simulink model "ExperimentalCarrier"  (R2015b)
settings: Solver=ode45  StartTime=0.0  StopTime=60  FixedStep=0.001  RelTol=1e-4
model workspace (MAT data in the model file):
  CX = [-0.0973267994662 -0.079334770792 -0.063312708602 -0.0492783817904 -0.0372483838751 -0.0272381795582 -0.0192622767468 -0.0133348794834 -0.00947247058383 -0.00770460619817 -0.00779177365154 -0.010332184952 ... (651 elements, 31x21)]
  CX_P = [0.00223913348595 0.00226279846593 0.00215584206323 0.00191826427785 0.0015500651098 0.00105124455907 0.000421802625665 -0.000338260690416 -0.00122894538917 -0.00225025147061 -0.00340217893471 -0.0046847277815 ... (651 elements, 31x21)]
  CX_Q = [0.566750126524 0.513799273419 0.46074149597 0.407560115115 0.354235092058 0.300738098816 0.247021798665 0.193002362465 0.138579422321 0.0841448328254 0.0156800910173 -0.028587220216 ... (651 elements, 31x21)]
  CX_R = [0.00872473439328 0.00961108484928 0.0104908055113 0.0113660862689 0.0122394567236 0.0131139410899 0.0139934759578 0.0148843304351 0.0158005787982 0.0167844985256 0.0173214701743 0.0192824833308 ... (651 elements, 31x21)]
  CX_d_elevator = [0.029681120923 0.0264274948833 0.0231424780296 0.019826833889 0.0164811360769 0.0131055318554 0.00969907215747 0.00625794011772 0.00277062099267 -0.000820697586383 -0.00752061307428 -0.00815142995882 ... (651 elements, 31x21)]
  CX_d_rudder = [-0.00683814731464 -0.00579287968011 -0.00473313798197 -0.00365917618136 -0.00257115069818 -0.00146908461552 -0.000352779652782 0.000778396676178 0.0019254949791 0.00307845824922 0.00430777388103 0.00587395376473 ... (651 elements, 31x21)]
  CY = [0.0748502535538 0.0755645920384 0.0762601803819 0.076936530444 0.0775935707011 0.0782321665355 0.078855460083 0.0794722913019 0.0801051244106 0.0807983900173 0.0815089407636 0.0810999911453 ... (651 elements, 31x21)]
  CY_P = [0.314314541533 0.314908852342 0.315908686179 0.317314043043 0.319124922936 0.321341325856 0.323963251804 0.32699070078 0.330423672784 0.334262167815 0.338506185874 0.343155726961 ... (651 elements, 31x21)]
  CY_Q = [0.206845108985 0.212153285689 0.217549246201 0.223041221006 0.22863865097 0.234352353828 0.240194164072 0.246174375163 0.252295596359 0.258590970539 0.26593702078 0.276814416222 ... (651 elements, 31x21)]
  CY_R = [-0.299983586918 -0.303050767939 -0.30608450573 -0.309088417238 -0.312066630946 -0.315024477354 -0.317970440697 -0.320921537604 -0.323916102322 -0.327010675103 -0.329661903523 -0.331314720608 ... (651 elements, 31x21)]
  CY_d_elevator = [0.0241602483601 0.024862141616 0.0255735782381 0.0262950172254 0.0270270636195 0.0277705820366 0.0285269750226 0.0292988478742 0.0300914026037 0.030913435532 0.0317596917419 0.0324941126108 ... (651 elements, 31x21)]
  CY_d_rudder = [-0.129392052709 -0.131156233114 -0.132888496587 -0.13458992916 -0.13626179938 -0.137905650351 -0.139523580046 -0.141119005177 -0.142698155317 -0.144262742569 -0.145575423934 -0.146927528452 ... (651 elements, 31x21)]
  CZ = [-0.635288026255 -0.561513437672 -0.486937541039 -0.411613157493 -0.335593450001 -0.258932000134 -0.181683022099 -0.10390236702 -0.025657439009 0.0528154193638 0.128636653723 0.209168379022 ... (651 elements, 31x21)]
  CZ_P = [-0.0426180741921 -0.040371283283 -0.0379977363135 -0.0354974332835 -0.0328703741931 -0.0301165590423 -0.027235987831 -0.0242286605594 -0.0210945772272 -0.0178337378347 -0.0144461423817 -0.0109317908683 ... (651 elements, 31x21)]
  CZ_Q = [6.96025865077 6.98114129849 7.00206820292 7.02304903766 7.04409127039 7.06519952703 7.08637371713 7.10760603499 7.12891815552 7.15129935899 7.15392062661 7.18837906802 ... (651 elements, 31x21)]
  CZ_R = [-0.105405414656 -0.106545289739 -0.107737293614 -0.108987554898 -0.110302712806 -0.111690005069 -0.113157533015 -0.114714527104 -0.116362189514 -0.11786971515 -0.114666901886 -0.118318379275 ... (651 elements, 31x21)]
  CZ_d_elevator = [0.51008994796 0.512918903365 0.515635142398 0.518238988463 0.520730557555 0.523109824579 0.525376856974 0.527532585768 0.529582683355 0.53158310039 0.53222009415 0.532991323176 ... (651 elements, 31x21)]
  CZ_d_rudder = [-0.0994246348718 -0.101114338005 -0.102795749856 -0.104468657243 -0.106132886268 -0.107788391525 -0.109435540346 -0.111075916846 -0.112714334729 -0.114363388416 -0.115472857798 -0.116943666826 ... (651 elements, 31x21)]
  Cl = [-0.0385814765962 -0.0383389644596 -0.0380848835968 -0.0378195009591 -0.0375431159662 -0.0372560730473 -0.0369588021987 -0.0366519368415 -0.0363364206354 -0.0360097812088 -0.0355885143095 -0.0352015390645 ... (651 elements, 31x21)]
  Cl_P = [-0.410096776624 -0.411715869817 -0.413321511523 -0.414913701743 -0.416492440476 -0.418057727723 -0.419609563483 -0.421147947757 -0.422672880544 -0.424184361845 -0.425682391659 -0.427166969987 ... (651 elements, 31x21)]
  Cl_Q = [0.0121734873015 0.0115511634771 0.0109219874117 0.0102856172191 0.00964162351347 0.00898936687588 0.00832771640535 0.00765433243871 0.00696211625156 0.00619409954578 0.00511750960358 0.00438446572798 ... (651 elements, 31x21)]
  Cl_R = [0.0639194118456 0.0641980766094 0.0644722880685 0.0647423901469 0.0650087480028 0.0652717875848 0.0655321272397 0.0657909713502 0.0660509927516 0.066314134037 0.0664428977346 0.0665956593355 ... (651 elements, 31x21)]
  Cl_d_elevator = [-0.00083845092376 -0.000897333841468 -0.000957239499541 -0.00101816580014 -0.00108011314323 -0.00114310126406 -0.00120721661945 -0.00127274325287 -0.00134057483614 -0.00141463059496 -0.00150116458646 -0.00150417720092 ... (651 elements, 31x21)]
  Cl_d_rudder = [0.0120074370195 0.0121224981409 0.0122343776715 0.0123431699853 0.0124489831282 0.0125519544191 0.0126522973225 0.0127504304685 0.0128472820476 0.012944583953 0.0130167454048 0.0130728202844 ... (651 elements, 31x21)]
  Cm = [0.0973465601848 0.0882383997807 0.0791321401801 0.0700083578182 0.060846163509 0.0516235998805 0.0423185376691 0.03291173616 0.0234098703618 0.0141912971055 0.0115389891247 -0.00108731819606 ... (651 elements, 31x21)]
  Cm_P = [0.204940910369 0.202805913545 0.20033190145 0.197518874086 0.194366831451 0.190875773546 0.187045700371 0.182876611925 0.17836850821 0.173521389224 0.168335254967 0.162810105441 ... (651 elements, 31x21)]
  Cm_Q = [-8.8302811579 -8.84673802608 -8.86380445529 -8.8815160128 -8.89990381522 -8.91899396376 -8.93880586357 -8.95935222087 -8.98073821097 -9.00528706826 -8.98625605481 -9.03648930164 ... (651 elements, 31x21)]
  Cm_R = [0.231203964913 0.23319997533 0.235299090374 0.237514849258 0.239861907942 0.242356170567 0.245015146547 0.247857975971 0.250885037596 0.253592063858 0.24580144055 0.252971901877 ... (651 elements, 31x21)]
  Cm_d_elevator = [-1.16934045694 -1.17556162403 -1.1814926709 -1.18713462751 -1.19248809506 -1.19755345312 -1.20233156667 -1.2068260282 -1.21105317786 -1.21514844284 -1.21623242778 -1.21673947768 ... (651 elements, 31x21)]
  Cm_d_rudder = [0.221327907125 0.224938352672 0.228521302045 0.232076418337 0.235603478751 0.239102604189 0.24257498777 0.246024952347 0.249465016904 0.252925369172 0.255135515483 0.258069205799 ... (651 elements, 31x21)]
  Cn = [0.0239084920706 0.0233651881183 0.0228219583067 0.0222793256831 0.0217379864069 0.0211990203144 0.0206644263801 0.0201384574022 0.0196305829364 0.0191582088364 0.0187126782059 0.0177875778536 ... (651 elements, 31x21)]
  Cn_P = [0.00271348744888 0.000830692215513 -0.000879092281498 -0.00241586604216 -0.00377962906647 -0.00497038135443 -0.00598812290603 -0.00683285372129 -0.0075045738002 -0.00800328314275 -0.00832898174895 -0.0084816696188 ... (651 elements, 31x21)]
  Cn_Q = [0.0646895607463 0.0668587351559 0.0690696353792 0.0713263026419 0.0736328941188 0.0759930959236 0.078408543068 0.0808750323066 0.0833760949483 0.0858871158776 0.0879312223138 0.0933690960242 ... (651 elements, 31x21)]
  Cn_R = [-0.107505906228 -0.108368888514 -0.109223762874 -0.110071896296 -0.110914888897 -0.111754897972 -0.112595502998 -0.113443913399 -0.114315599189 -0.115230945783 -0.115971844659 -0.116177724127 ... (651 elements, 31x21)]
  Cn_d_elevator = [0.00836627067687 0.00863561072168 0.00890974810625 0.00918895143726 0.009473528048 0.00976381947702 0.0100601758992 0.0103628424776 0.0106713097064 0.0109780163579 0.011109463637 0.0115746093706 ... (651 elements, 31x21)]
  Cn_d_rudder = [-0.0546400598137 -0.0553510121202 -0.0560495856635 -0.0567362885882 -0.0574116958811 -0.0580764807608 -0.0587315154598 -0.0593781486964 -0.060018716409 -0.060653217797 -0.0611661774955 -0.061673059209 ... (651 elements, 31x21)]
  aircraft_geometry_name = 'ExperimentalCarrier'
  alpha = [-0.174532925199 -0.157079632679 -0.13962634016 -0.12217304764 -0.10471975512 -0.0872664625997 -0.0698131700798 -0.0523598775598 -0.0349065850399 -0.0174532925199 0 0.0174532925199 ... (31 elements, 31x1)]
  beta = [-0.174532925199 -0.157079632679 -0.13962634016 -0.12217304764 -0.10471975512 -0.0872664625997 -0.0698131700798 -0.0523598775598 -0.0349065850399 -0.0174532925199 0 0.0174532925199 ... (21 elements, 21x1)]
  centerOfGravity = -0.092
  mass = 1.56
  mean_chord = 0.25
  spanwidth = 1.5
undefined symbols (not defined in the file): Earth, WGS84
libraries: aerolibconvert2 x6, aerolibnav x3, aerolibasang x2, aerolibfltsims x2, aerolib6dof2 x1, aerolibadyn x1, aerolibtransform2 x1, aerolibanimutils x1, aerolibatmos2 x1, aerolibgravity2 x1
(part 2 of 2)

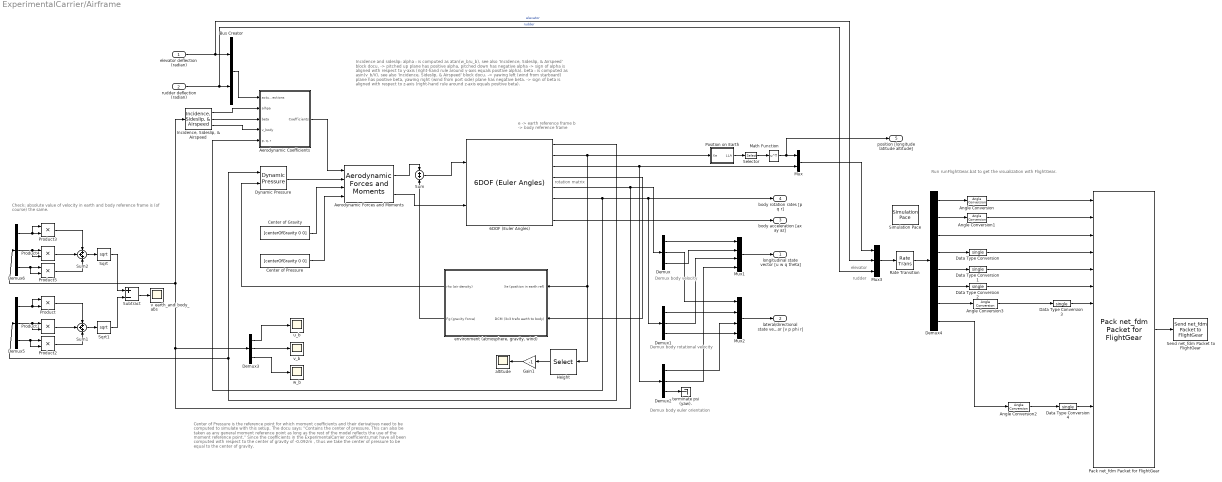
== system ExperimentalCarrier/Airframe ==
  note: rotation matrix
  note: Check: absolute value of velocity in earth and body reference frame is
      | (of course) the same.
  note: rudder
  note: elevator
  note: Incidence and sideslip:
      | alpha : is computed as atan(w_b/u_b), see also 'Incidence, Sideslip, & Airspeed' block docu.
      | -> pitched up plane has positive alpha, pitched down has negative alpha
      | -> sign of alpha is aligned with respect to y-axis (right-hand rule around y-axis equals positive alpha).
      | beta : is computed as asin(v_b/V), see also 'Incidence, Sideslip, & Airspeed' block docu.
      | -> yawing left (wind from starboard) plane has positive beta, yawing right (wind from port side) plane has negative beta.
      | -> sign of beta is aligned with respect to z-axis (right-hand rule around z-axis equals positive beta).
  note: Demux body velocity
  note: Run runFlightGear.bat to get the visualization with FlightGear.
  note: e -> earth reference frame
      | b -> body reference frame
  note: Center of Pressure is the reference point for which moment coefficients and their derivatives need to be computed to simulate with this setup.
      | The docu says: "Contains the center of pressure. This can also be taken as any general moment reference point as long as the rest of the model
      | reflects the use of the moment reference point." Since the coefficients in the ExperimentalCarrier coefficients.mat have all been computed with respect to
      | the center of gravity of -0.092m , thus we take the center of pressure to be equal to the center of gravity.
  note: Demux body rotational velocity
  note: Demux body euler orientation
  elevator deflection (radian) : Inport
  rudder deflection (radian) : Inport  Port=2
  6DOF (Euler Angles) : aerolib6dof2/6DOF (Euler Angles)  units=Metric (MKS)  mtype=Fixed  rep=Euler Angles  xme_0=[-12071.91150883141;0;-800.0]  Vm_0=[11 0 0]  eul_0=[0 -1.2 0]  pm_0=[0 0 0]  mass_0=mass  mass_e=0.5  mass_f=2.0  inertia=eye(3)  inertia_e=eye(3)  inertia_f=2*eye(3)  k_quat=1.0  vre_flag=on
  "Aerodynamic Forces and Moments " : aerolibadyn/Aerodynamic Forces and Moments   inputAxes=Body  outputForceAxes=Body  outputMomentAxes=Body  S=spanwidth*mean_chord  b=spanwidth  cbar=mean_chord
  Aerodynamic Coefficients : Subsystem
  Angle Conversion : aerolibconvert2/Angle Conversion  IU=deg  OU=rad
  Angle Conversion1 : aerolibconvert2/Angle Conversion  IU=deg  OU=rad
  Angle Conversion2 : aerolibconvert2/Angle Conversion  IU=rad  OU=deg
  Angle Conversion3 : aerolibconvert2/Angle Conversion  IU=rad  OU=deg
  Bus Creator : BusCreator  Inputs=2
  Center of Gravity : Constant  Value=[centerOfGravity 0 0]
  Center of Pressure : Constant  Value=[centerOfGravity 0 0]
  Data Type Conversion{,1..4} (5 alike) : DataTypeConversion  OutDataTypeStr=single
  Demux{,1..3,5..6} (6 alike) : Demux  Outputs=3
  Demux4 : Demux  Outputs=8
  Dynamic Pressure : aerolibasang/Dynamic Pressure
  Gain1 : Gain  Gain=-1
  Height : Selector  InputPortWidth=3  IndexOptions=Index vector (dialog)  Indices=[3]  OutputSizes=1
  "Incidence, Sideslip, & Airspeed" : aerolibasang/Incidence, Sideslip, & Airspeed
  Math Function : Math  Operator=transpose  SaturateOnIntegerOverflow=on
  Mux : Mux  Inputs=2
  Mux1 : Mux
  Mux2 : Mux
  Mux3 : Mux  Inputs=3
  Pack net_fdm Packet for FlightGear : aerolibfltsims/Pack net_fdm Packet for FlightGear  FlightGearVersion=v3.4  ShowPositionAttitudeInputs=on  ShowVelocityAccelerationInputs=off  ShowControlSurfacePositionInputs=on  ShowEngineFuelInputs=off  ShowLandingGearInputs=off  ShowEnvironmentInputs=off  SampleTime=1/30
  Position on Earth : Subsystem  Priority=1  TreatAsAtomicUnit=on
  Product{,1..5} (6 alike) : Product  RndMeth=Zero
  Rate Transition : RateTransition  Integrity=off  OutPortSampleTime=1/30
  Selector : Selector  InputPortWidth=3  IndexOptions=Index vector (dialog)  Indices=[2 1 3]  OutputSizes=1
  Send net_fdm Packet to FlightGear : aerolibfltsims/Send net_fdm Packet to FlightGear  DestinationIpAddress=127.0.0.1  DestinationPort=5502  LocalIpPort=-1  varLen=off  SampleTime=1/30
  Simulation Pace : aerolibanimutils/Simulation Pace  SimulationPace=1  SleepMode=MATLAB Thread  OutputPaceError=off  SampleTime=1/30
      settings: AttributesFormatString=%<SimulationPace> sec/sec
  Sqrt : Sqrt  SaturateOnIntegerOverflow=on
  Sqrt1 : Sqrt  SaturateOnIntegerOverflow=on
  Subtract : Sum  Inputs=+-
  Sum : Sum
  Sum1 : Sum  Inputs=+++
  Sum2 : Sum  Inputs=+++
  altitude : Scope
  "environment (atmosphere, gravity, wind)" : Subsystem
  terminate psi (yaw). : Terminator
  u_b : Scope
  v_b : Scope
  v_earth_and_body_abs : Scope
  w_b : Scope
  longitudinal state vector [u w q theta] : Outport
  lateral/directional state vector [v p phi r] : Outport  Port=2
  body acceleration [ax ay az] : Outport  Port=3
  body rotation rates [p q r] : Outport  Port=4
  position [longitude latitude altitude] : Outport  Port=5
  wires:
  "Aerodynamic Forces and Moments "/1 -> Sum/1
  "Aerodynamic Forces and Moments "/2 -> 6DOF (Euler Angles)/2
  Center of Gravity/1 -> "Aerodynamic Forces and Moments "/3
  Center of Pressure/1 -> "Aerodynamic Forces and Moments "/4
  Dynamic Pressure/1 -> "Aerodynamic Forces and Moments "/2
  6DOF (Euler Angles)/1 -> Dynamic Pressure/1, Demux5/1
  6DOF (Euler Angles)/2 -> Height/1, "environment (atmosphere, gravity, wind)"/1(Xe (position in earth ref)), Position on Earth/1(Xe)
  Position on Earth/1(LLA) -> Selector/1
  6DOF (Euler Angles)/4 -> "environment (atmosphere, gravity, wind)"/2(DCM (3x3 trafo earth to body))
  6DOF (Euler Angles)/3 -> Mux/2, Demux2/1
  6DOF (Euler Angles)/5 -> "Incidence, Sideslip, & Airspeed"/1, Demux6/1, Demux3/1, Demux/1
  6DOF (Euler Angles)/6 -> Aerodynamic Coefficients/5("p, q, r"), body rotation rates [p q r]/1, Demux1/1
  Math Function/1 -> position [longitude latitude altitude]/1, Mux/1
  Mux/1 -> Mux3/1
  Selector/1 -> Math Function/1
  "environment (atmosphere, gravity, wind)"/1(rho (air density)) -> Dynamic Pressure/2
  "environment (atmosphere, gravity, wind)"/2(Fg (gravity force)) -> Sum/2
  Height/1 -> Gain1/1
  "Incidence, Sideslip, & Airspeed"/1 -> Aerodynamic Coefficients/2(alhpa)
  "Incidence, Sideslip, & Airspeed"/2 -> Aerodynamic Coefficients/3(beta)
  "Incidence, Sideslip, & Airspeed"/3 -> Aerodynamic Coefficients/4(v_body)
  Aerodynamic Coefficients/1(Coefficients) -> "Aerodynamic Forces and Moments "/1
  Gain1/1 -> altitude/1
  Bus Creator/1 -> Aerodynamic Coefficients/1(actuator deflections)
  elevator deflection (radian)/1 -> Mux3/2, Bus Creator/1  "elevator"
  rudder deflection (radian)/1 -> Mux3/3, Bus Creator/2  "rudder"
  Sum/1 -> 6DOF (Euler Angles)/1
  Demux/1 -> Mux1/1
  Demux/3 -> Mux1/2
  Demux/2 -> Mux2/1
  Demux1/2 -> Mux1/3
  Demux1/1 -> Mux2/2
  Demux1/3 -> Mux2/4
  Demux2/1 -> Mux2/3
  Demux2/2 -> Mux1/4
  Demux2/3 -> terminate psi (yaw)./1
  Mux2/1 -> lateral/directional state vector [v p phi r]/1
  Mux1/1 -> longitudinal state vector [u w q theta]/1
  Demux3/1 -> u_b/1
  Demux3/2 -> v_b/1
  Demux3/3 -> w_b/1
  Pack net_fdm Packet for FlightGear/1 -> Send net_fdm Packet to FlightGear/1
  Demux4/1 -> Angle Conversion/1
  Demux4/2 -> Angle Conversion1/1
  Demux4/3 -> Pack net_fdm Packet for FlightGear/3
  Demux4/4 -> Data Type Conversion/1
  Demux4/5 -> Data Type Conversion1/1
  Demux4/6 -> Data Type Conversion2/1
  Rate Transition/1 -> Demux4/1
  Angle Conversion/1 -> Pack net_fdm Packet for FlightGear/1
  Angle Conversion1/1 -> Pack net_fdm Packet for FlightGear/2
  Data Type Conversion/1 -> Pack net_fdm Packet for FlightGear/4
  Data Type Conversion1/1 -> Pack net_fdm Packet for FlightGear/5
  Data Type Conversion2/1 -> Pack net_fdm Packet for FlightGear/6
  Mux3/1 -> Rate Transition/1
  Demux4/7 -> Angle Conversion3/1
  Demux4/8 -> Angle Conversion2/1
  Data Type Conversion3/1 -> Pack net_fdm Packet for FlightGear/7
  Data Type Conversion4/1 -> Pack net_fdm Packet for FlightGear/13
  Angle Conversion2/1 -> Data Type Conversion4/1
  Angle Conversion3/1 -> Data Type Conversion3/1
  Product2/1 -> Sum1/3
  Demux5/3 -> Product2/2, Product2/1
  Product/1 -> Sum1/1
  Product1/1 -> Sum1/2
  Sum1/1 -> Sqrt1/1
  Demux5/1 -> Product/2, Product/1
  Demux5/2 -> Product1/1, Product1/2
  Product5/1 -> Sum2/3
  Demux6/3 -> Product5/2, Product5/1
  Product3/1 -> Sum2/1
  Product4/1 -> Sum2/2
  Sum2/1 -> Sqrt/1
  Demux6/1 -> Product3/2, Product3/1
  Demux6/2 -> Product4/1, Product4/2
  Sqrt/1 -> Subtract/1
  Sqrt1/1 -> Subtract/2
  Subtract/1 -> v_earth_and_body_abs/1
  6DOF (Euler Angles)/8 -> body acceleration [ax ay az]/1

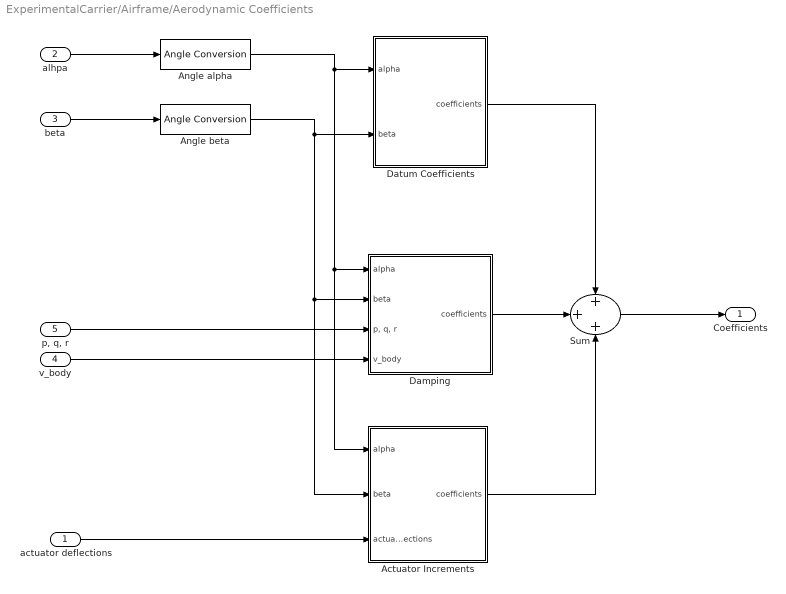
== system ExperimentalCarrier/Airframe/Aerodynamic Coefficients ==
  actuator deflections : Inport
  alhpa : Inport  Port=2
  beta : Inport  Port=3
  v_body : Inport  Port=4
  "p, q, r" : Inport  Port=5
  Actuator Increments : Subsystem
  Angle alpha : aerolibconvert2/Angle Conversion  IU=rad  OU=deg
  Angle beta : aerolibconvert2/Angle Conversion  IU=rad  OU=deg
  Damping : Subsystem
  Datum Coefficients : Subsystem
  Sum : Sum  Inputs=+++
  Coefficients : Outport
  wires:
  alhpa/1 -> Angle alpha/1
  Angle alpha/1 -> Actuator Increments/1(alpha), Damping/1(alpha), Datum Coefficients/1(alpha)
  Angle beta/1 -> Actuator Increments/2(beta), Damping/2(beta), Datum Coefficients/2(beta)
  Datum Coefficients/1(coefficients) -> Sum/1
  "p, q, r"/1 -> Damping/3("p, q, r")
  Damping/1(coefficients) -> Sum/2
  Sum/1 -> Coefficients/1
  v_body/1 -> Damping/4(v_body)
  beta/1 -> Angle beta/1
  actuator deflections/1 -> Actuator Increments/3(actuator deflections)
  Actuator Increments/1(coefficients) -> Sum/3

== system ExperimentalCarrier/Airframe/Position on Earth ==
  Xe : Inport
  Flat Earth to LLA : aerolibtransform2/Flat Earth to LLA  units=Metric (MKS)  ptype=Earth (WGS84)  F=1/298.257223563  R=6378137  LL0=[37.628738616666666,-1.223933911333333e+02]  psi=0
  Mux : Mux  Inputs=2
  href : Constant  Value=300
  LLA : Outport
  wires:
  Mux/1 -> LLA/1
  Xe/1 -> Flat Earth to LLA/1
  Flat Earth to LLA/1 -> Mux/1
  Flat Earth to LLA/2 -> Mux/2
  href/1 -> Flat Earth to LLA/2

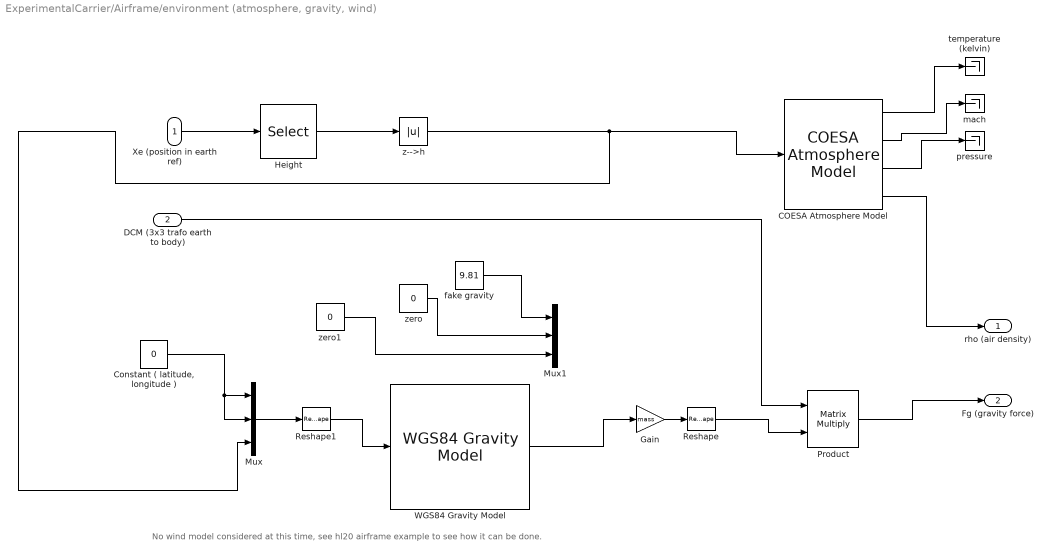
== system ExperimentalCarrier/Airframe/environment (atmosphere, gravity, wind) ==
  note: No wind model considered at this time, see hl20 airframe example to see how it can be done.
  Xe (position in earth ref) : Inport
  DCM (3x3 trafo earth to body) : Inport  Port=2
  COESA Atmosphere Model : aerolibatmos2/COESA Atmosphere Model  units=Metric (MKS)  spec=1976 COESA-extended U.S. Standard Atmosphere  model=Profile  profile_var=High temperature  profile_percent=1%  profile_alt=5 km (16404 ft)  envelope_var=High temperature  envelope_percent=1%  action=Warning
  "Constant ( latitude, longitude )" : Constant  Value=0
  Gain : Gain  Gain=mass
  Height : Selector  InputPortWidth=3  IndexOptions=Index vector (dialog)  Indices=[3]  OutputSizes=1
  Mux : Mux  Inputs=3
  Mux1 : Mux  Inputs=3
  Product : Product  Multiplication=Matrix(*)
  Reshape : Reshape
  Reshape1 : Reshape
  "WGS84 Gravity Model " : aerolibgravity2/WGS84 Gravity Model   model=WGS84 Taylor Series  units=Metric (MKS)  no_atmos=on  precessing=on  jd_loc=off  month=October  day=10  year=2004  no_centrifugal=on  action=Warning
  fake gravity : Constant  Value=9.81
  mach : Terminator
  pressure : Terminator
  temperature (kelvin) : Terminator
  z-->h : Abs  SaturateOnIntegerOverflow=on
  zero : Constant  Value=0
  zero1 : Constant  Value=0
  rho (air density) : Outport
  Fg (gravity force) : Outport  Port=2
  wires:
  Xe (position in earth ref)/1 -> Height/1
  Height/1 -> z-->h/1
  z-->h/1 -> Mux/3, COESA Atmosphere Model/1
  COESA Atmosphere Model/4 -> rho (air density)/1
  COESA Atmosphere Model/1 -> temperature (kelvin)/1
  COESA Atmosphere Model/2 -> mach/1
  COESA Atmosphere Model/3 -> pressure/1
  "Constant ( latitude, longitude )"/1 -> Mux/1, Mux/2
  Mux/1 -> Reshape1/1
  fake gravity/1 -> Mux1/1
  Gain/1 -> Reshape/1
  Reshape/1 -> Product/2
  DCM (3x3 trafo earth to body)/1 -> Product/1
  Product/1 -> Fg (gravity force)/1
  zero/1 -> Mux1/2
  zero1/1 -> Mux1/3
  Reshape1/1 -> "WGS84 Gravity Model "/1
  "WGS84 Gravity Model "/1 -> Gain/1

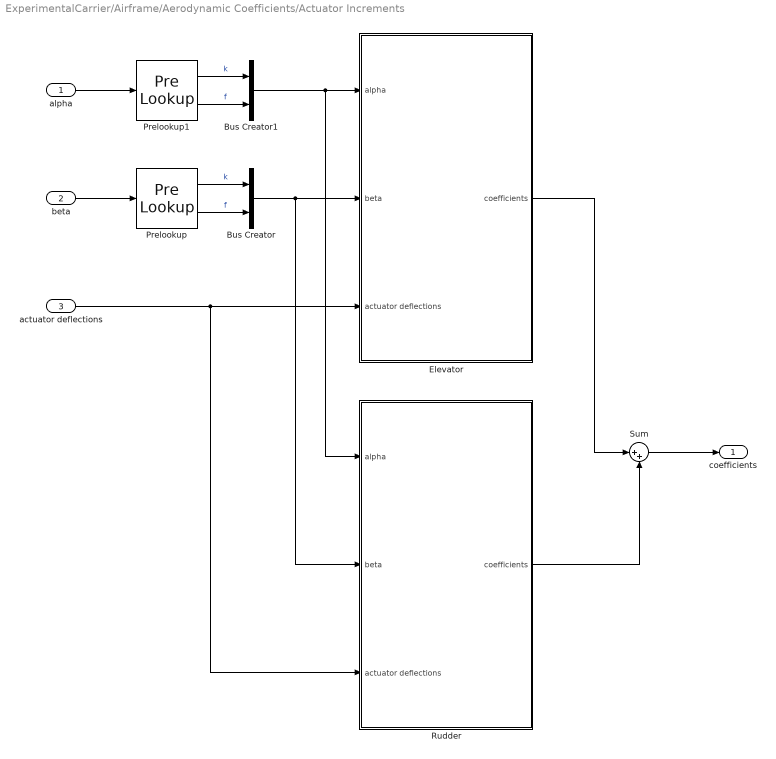
== system ExperimentalCarrier/Airframe/Aerodynamic Coefficients/Actuator Increments ==
  alpha : Inport
  beta : Inport  Port=2
  actuator deflections : Inport  Port=3
  Bus Creator : BusCreator  Inputs=2
  Bus Creator1 : BusCreator  Inputs=2
  Elevator : Subsystem
  Prelookup : PreLookup  BreakpointsData=beta*180/pi  ExtrapMethod=Linear
  Prelookup1 : PreLookup  BreakpointsData=alpha*180/pi  ExtrapMethod=Linear
  Rudder : Subsystem
  Sum : Sum  Inputs=|++
  coefficients : Outport
  wires:
  alpha/1 -> Prelookup1/1
  beta/1 -> Prelookup/1
  actuator deflections/1 -> Rudder/3(actuator deflections), Elevator/3(actuator deflections)
  Elevator/1(coefficients) -> Sum/1
  Sum/1 -> coefficients/1
  Bus Creator/1 -> Elevator/2(beta), Rudder/2(beta)
  Prelookup/1 -> Bus Creator/1  "k"
  Prelookup/2 -> Bus Creator/2  "f"
  Prelookup1/1 -> Bus Creator1/1  "k"
  Prelookup1/2 -> Bus Creator1/2  "f"
  Bus Creator1/1 -> Elevator/1(alpha), Rudder/1(alpha)
  Rudder/1(coefficients) -> Sum/2

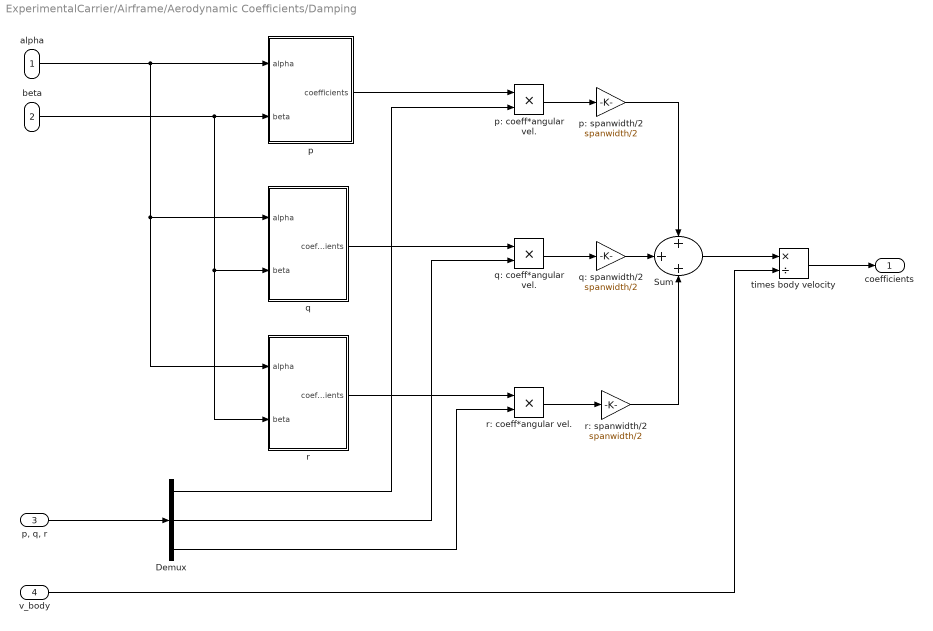
== system ExperimentalCarrier/Airframe/Aerodynamic Coefficients/Damping ==
  alpha : Inport
  beta : Inport  Port=2
  "p, q, r" : Inport  Port=3
  v_body : Inport  Port=4
  Demux : Demux  Outputs=3
  Sum : Sum  Inputs=+++
  p : Subsystem
  p: coeff*angular vel. : Product
  p: spanwidth/2 : Gain  Gain=spanwidth/2
  q : Subsystem
  q: coeff*angular vel. : Product
  q: spanwidth/2 : Gain  Gain=spanwidth/2
  r : Subsystem
  r: coeff*angular vel. : Product
  r: spanwidth/2 : Gain  Gain=spanwidth/2
  times body velocity : Product  Inputs=*/
  coefficients : Outport
  wires:
  alpha/1 -> r/1(alpha), q/1(alpha), p/1(alpha)
  beta/1 -> r/2(beta), q/2(beta), p/2(beta)
  p/1(coefficients) -> p: coeff*angular vel./1
  "p, q, r"/1 -> Demux/1
  p: coeff*angular vel./1 -> p: spanwidth/2/1
  p: spanwidth/2/1 -> Sum/1
  Sum/1 -> times body velocity/1
  v_body/1 -> times body velocity/2
  q/1(coefficients) -> q: coeff*angular vel./1
  r/1(coefficients) -> r: coeff*angular vel./1
  q: spanwidth/2/1 -> Sum/2
  r: spanwidth/2/1 -> Sum/3
  r: coeff*angular vel./1 -> r: spanwidth/2/1
  q: coeff*angular vel./1 -> q: spanwidth/2/1
  Demux/2 -> q: coeff*angular vel./2
  times body velocity/1 -> coefficients/1
  Demux/1 -> p: coeff*angular vel./2
  Demux/3 -> r: coeff*angular vel./2

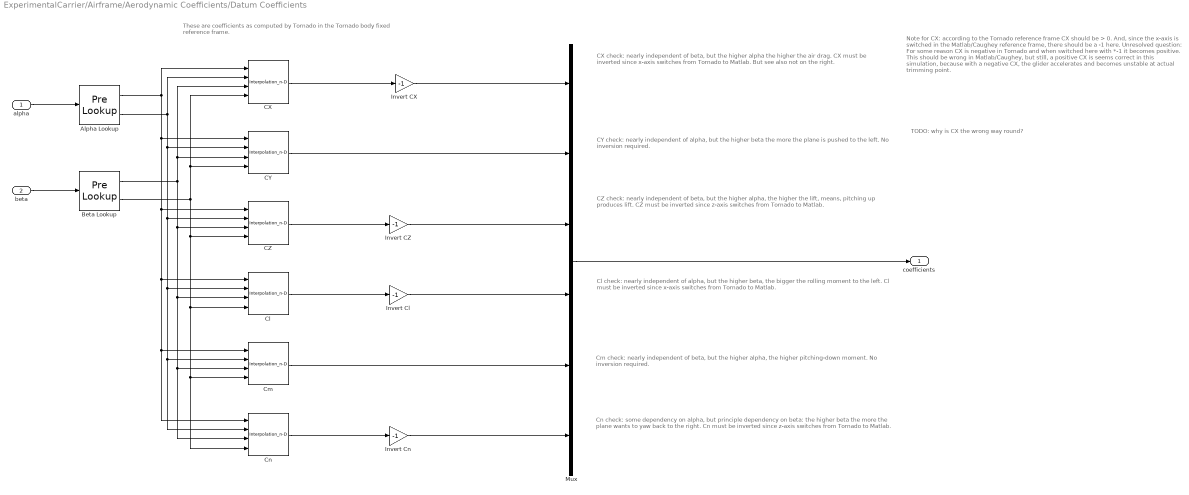
== system ExperimentalCarrier/Airframe/Aerodynamic Coefficients/Datum Coefficients ==
  note: Cl check: nearly independent of alpha, but the higher beta, the bigger the rolling moment to the left. Cl must be inverted since x-axis switches from Tornado to Matlab.
  note: CY check: nearly independent of alpha, but
      | the higher beta the more the plane is pushed to the left. No inversion required.
  note: These are coefficients as computed by Tornado in the
      | Tornado body fixed reference frame.
  note: Cm check: nearly independent of beta, but the higher alpha, the higher pitching-down moment. No inversion required.
  note: CZ check: nearly independent of beta, but the higher alpha, the higher the lift, means, pitching up produces lift. CZ must be inverted since z-axis switches from Tornado to Matlab.
  note: Note for CX: according to the Tornado reference frame
      | CX should be > 0. And, since the x-axis is switched in the
      | Matlab/Caughey reference frame, there should be a -1 here.
      | Unresolved question: For some reason CX is negative in Tornado
      | and when switched here with *-1 it becomes positive. This should
      | be wrong in Matlab/Caughey, but still, a positive CX is seems correct
      | in this simulation, because with a negative CX, the glider
      | accelerates and becomes unstable at actual trimming point.
  note: Cn check: some dependency on alpha, but principle dependency on beta: the higher beta the more the plane wants to yaw back to the right. Cn must be inverted since z-axis switches from Tornado to Matlab.
  note: CX check: nearly independent of beta, but the higher alpha the higher the air drag. CX must be inverted since x-axis switches from Tornado to Matlab. But see also not on the right.
  note: TODO:
      | why is CX the wrong way round?
  alpha : Inport
  beta : Inport  Port=2
  Alpha Lookup : PreLookup  BreakpointsData=alpha*180/pi  ExtrapMethod=Linear
  Beta Lookup : PreLookup  BreakpointsData=beta*180/pi  ExtrapMethod=Linear
  CX : Interpolation_n-D  Table=CX  InternalRulePriority=Speed
  CY : Interpolation_n-D  Table=CY  InternalRulePriority=Speed
  CZ : Interpolation_n-D  Table=CZ  InternalRulePriority=Speed
  Cl : Interpolation_n-D  Table=Cl  InternalRulePriority=Speed
  Cm : Interpolation_n-D  Table=Cm  InternalRulePriority=Speed
  Cn : Interpolation_n-D  Table=Cn  InternalRulePriority=Speed
  Invert CX : Gain  Gain=-1
  Invert CZ : Gain  Gain=-1
  Invert Cl : Gain  Gain=-1
  Invert Cn : Gain  Gain=-1
  Mux : Mux  Inputs=6
  coefficients : Outport
  wires:
  Alpha Lookup/1 -> Cl/1, Cm/1, Cn/1, CZ/1, CY/1, CX/1
  Alpha Lookup/2 -> Cm/2, Cn/2, Cl/2, CZ/2, CY/2, CX/2
  Beta Lookup/1 -> Cn/3, Cm/3, Cl/3, CZ/3, CX/3, CY/3
  Beta Lookup/2 -> Cm/4, Cn/4, Cl/4, CZ/4, CX/4, CY/4
  alpha/1 -> Alpha Lookup/1
  beta/1 -> Beta Lookup/1
  Mux/1 -> coefficients/1
  CZ/1 -> Invert CZ/1
  CY/1 -> Mux/2
  CX/1 -> Invert CX/1
  Cl/1 -> Invert Cl/1
  Cn/1 -> Invert Cn/1
  Invert CZ/1 -> Mux/3
  Invert Cl/1 -> Mux/4
  Invert Cn/1 -> Mux/6
  Invert CX/1 -> Mux/1
  Cm/1 -> Mux/5

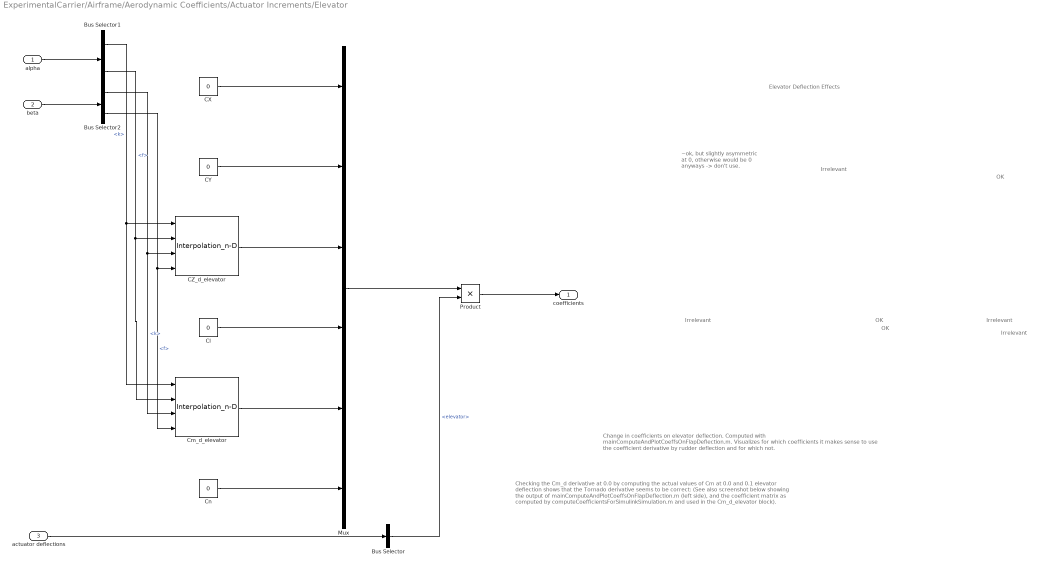
== system ExperimentalCarrier/Airframe/Aerodynamic Coefficients/Actuator Increments/Elevator ==
  note: Checking the Cm_d derivative at 0.0 by computing the actual values of Cm at 0.0 and 0.1 elevator deflection shows that the Tornado derivative seems to be correct:
      | (See also screenshot below showing the output of mainComputeAndPlotCoeffsOnFlapDeflection.m (left side), and the coefficient matrix as computed by computeCoefficientsForSimulinkSimulation.m and used in the Cm_d_elevator block).
  note: OK
  note: Irrelevant
  note: ~ok, but slightly
      | asymmetric at 0,
      | otherwise would
      | be 0 anyways
      | -> don't use.
  note: Irrelevant
  note: OK
  note: Irrelevant
  note: Change in coefficients on elevator deflection. Computed with mainComputeAndPlotCoeffsOnFlapDeflection.m.
      | Visualizes for which coefficients it makes sense to use the coefficient derivative by rudder deflection and for which not.
  note: Elevator Deflection Effects
  note: OK
  note: Irrelevant
  alpha : Inport
  beta : Inport  Port=2
  actuator deflections : Inport  Port=3
  Bus Selector : BusSelector  OutputSignals=elevator
  Bus Selector1 : BusSelector  OutputSignals=k,f
  Bus Selector2 : BusSelector  OutputSignals=k,f
  CX : Constant  Value=0
  CY : Constant  Value=0
  CZ_d_elevator : Interpolation_n-D  Table=CZ_d_elevator  InternalRulePriority=Speed
  Cl : Constant  Value=0
  Cm_d_elevator : Interpolation_n-D  Table=Cm_d_elevator  InternalRulePriority=Speed
  Cn : Constant  Value=0
  Mux : Mux  Inputs=6
  Product : Product
  coefficients : Outport
  wires:
  Bus Selector1/1 -> Cm_d_elevator/1, CZ_d_elevator/1  "<k>"
  Bus Selector1/2 -> Cm_d_elevator/2, CZ_d_elevator/2  "<f>"
  alpha/1 -> Bus Selector1/1
  Bus Selector2/1 -> Cm_d_elevator/3, CZ_d_elevator/3  "<k>"
  Bus Selector2/2 -> Cm_d_elevator/4, CZ_d_elevator/4  "<f>"
  CY/1 -> Mux/2
  CZ_d_elevator/1 -> Mux/3
  Cm_d_elevator/1 -> Mux/5
  actuator deflections/1 -> Bus Selector/1
  Product/1 -> coefficients/1
  Bus Selector/1 -> Product/2  "<elevator>"
  Mux/1 -> Product/1
  beta/1 -> Bus Selector2/1
  Cl/1 -> Mux/4
  Cn/1 -> Mux/6
  CX/1 -> Mux/1

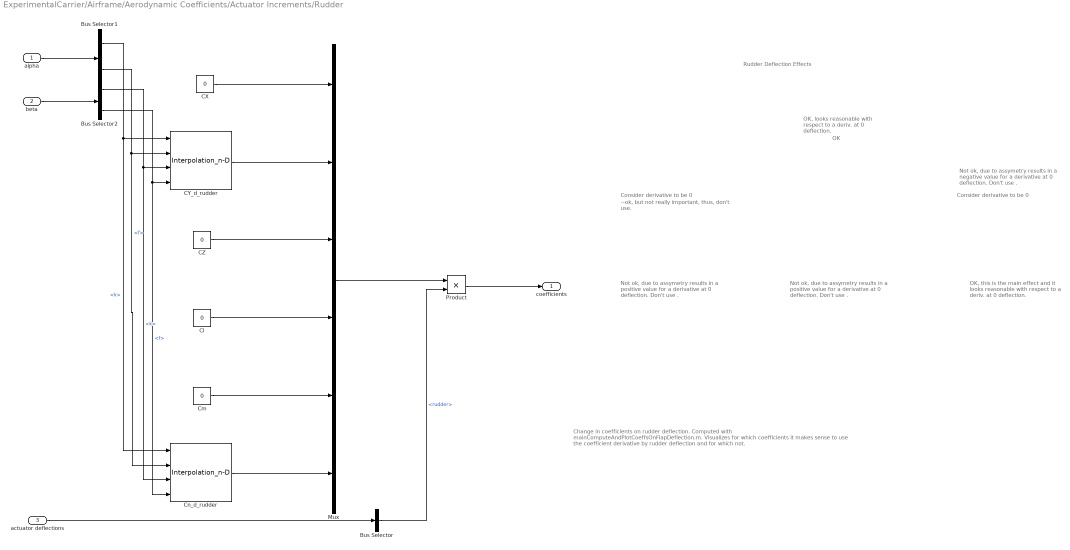
== system ExperimentalCarrier/Airframe/Aerodynamic Coefficients/Actuator Increments/Rudder ==
  note: Consider derivative to be 0
  note: Consider derivative to be 0
  note: OK
  note: Not ok, due to assymetry
      | results in a positive
      | value for a derivative at 0
      | deflection. Don't use .
  note: Not ok, due to assymetry
      | results in a positive
      | value for a derivative at 0
      | deflection. Don't use .
  note: OK, this is the main effect
      | and it looks reasonable
      | with respect to a deriv.
      | at 0 deflection.
  note: Not ok, due to assymetry
      | results in a negative
      | value for a derivative at 0
      | deflection. Don't use .
  note: OK, looks reasonable
      | with respect to a deriv.
      | at 0 deflection.
  note: ~ok, but not really important,
      | thus, don't use.
  note: Change in coefficients on rudder deflection. Computed with mainComputeAndPlotCoeffsOnFlapDeflection.m.
      | Visualizes for which coefficients it makes sense to use the coefficient derivative by rudder deflection and for which not.
  note: Rudder Deflection Effects
  alpha : Inport
  beta : Inport  Port=2
  actuator deflections : Inport  Port=3
  Bus Selector : BusSelector  OutputSignals=rudder
  Bus Selector1 : BusSelector  OutputSignals=k,f
  Bus Selector2 : BusSelector  OutputSignals=k,f
  CX : Constant  Value=0
  CY_d_rudder : Interpolation_n-D  Table=CY_d_rudder  InternalRulePriority=Speed
  CZ : Constant  Value=0
  Cl : Constant  Value=0
  Cm : Constant  Value=0
  Cn_d_rudder : Interpolation_n-D  Table=Cn_d_rudder  InternalRulePriority=Speed
  Mux : Mux  Inputs=6
  Product : Product
  coefficients : Outport
  wires:
  Bus Selector1/1 -> Cn_d_rudder/1, CY_d_rudder/1  "<k>"
  Bus Selector1/2 -> Cn_d_rudder/2, CY_d_rudder/2  "<f>"
  alpha/1 -> Bus Selector1/1
  Bus Selector2/1 -> Cn_d_rudder/3, CY_d_rudder/3  "<k>"
  Bus Selector2/2 -> Cn_d_rudder/4, CY_d_rudder/4  "<f>"
  CX/1 -> Mux/1
  CY_d_rudder/1 -> Mux/2
  CZ/1 -> Mux/3
  Cl/1 -> Mux/4
  Cn_d_rudder/1 -> Mux/6
  actuator deflections/1 -> Bus Selector/1
  Product/1 -> coefficients/1
  Bus Selector/1 -> Product/2  "<rudder>"
  Mux/1 -> Product/1
  beta/1 -> Bus Selector2/1
  Cm/1 -> Mux/5

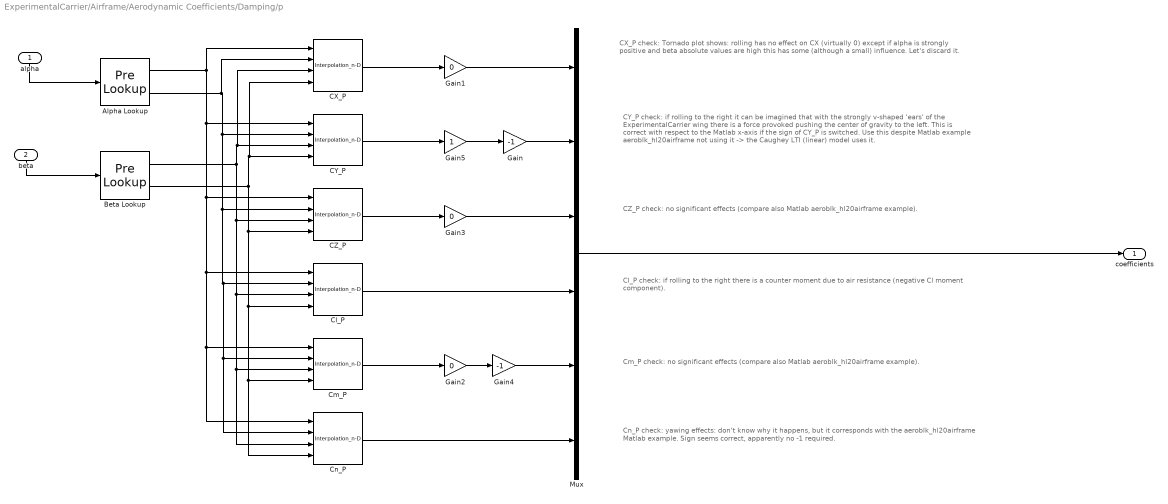
== system ExperimentalCarrier/Airframe/Aerodynamic Coefficients/Damping/p ==
  note: Cn_P check: yawing effects: don't know why it happens, but it corresponds with the aeroblk_hl20airframe Matlab example. Sign seems correct, apparently no -1 required.
  note: CZ_P check: no significant effects (compare also Matlab aeroblk_hl20airframe example).
  note: Cl_P check: if rolling to the right there is a counter moment due to air resistance (negative Cl moment component).
  note: CY_P check: if rolling to the right it can be imagined that with the strongly v-shaped 'ears' of the ExperimentalCarrier wing there is a force provoked pushing the center of gravity to the left. This is correct with respect to the Matlab x-axis if the sign of CY_P is switched. Use this despite Matlab example aeroblk_hl20airframe not using it -> the Caughey LTI (linear) model uses it.
  note: CX_P check: Tornado plot shows: rolling has no effect on CX (virtually 0) except if alpha is strongly positive and beta absolute values are high this has some (although a small) influence. Let's discard it.
  note: Cm_P check: no significant effects (compare also Matlab aeroblk_hl20airframe example).
  alpha : Inport
  beta : Inport  Port=2
  Alpha Lookup : PreLookup  BreakpointsData=alpha*180/pi  ExtrapMethod=Linear
  Beta Lookup : PreLookup  BreakpointsData=beta*180/pi  ExtrapMethod=Linear
  CX_P : Interpolation_n-D  Table=CX_P  InternalRulePriority=Speed
  CY_P : Interpolation_n-D  Table=CY_P  InternalRulePriority=Speed
  CZ_P : Interpolation_n-D  Table=CZ_P  InternalRulePriority=Speed
  Cl_P : Interpolation_n-D  Table=Cl_P  InternalRulePriority=Speed
  Cm_P : Interpolation_n-D  Table=Cm_P  InternalRulePriority=Speed
  Cn_P : Interpolation_n-D  Table=Cn_P  InternalRulePriority=Speed
  Gain : Gain  Gain=-1
  Gain1 : Gain  Gain=0
  Gain2 : Gain  Gain=0
  Gain3 : Gain  Gain=0
  Gain4 : Gain  Gain=-1
  Gain5 : Gain
  Mux : Mux  Inputs=6
  coefficients : Outport
  wires:
  Beta Lookup/2 -> CZ_P/4, Cn_P/4, Cm_P/4, Cl_P/4, CX_P/4, CY_P/4
  Alpha Lookup/1 -> CY_P/1, Cm_P/1, Cn_P/1, Cl_P/1, CZ_P/1, CX_P/1
  CX_P/1 -> Gain1/1
  Beta Lookup/1 -> CZ_P/3, Cn_P/3, Cm_P/3, Cl_P/3, CX_P/3, CY_P/3
  beta/1 -> Beta Lookup/1
  Alpha Lookup/2 -> CX_P/2, CY_P/2, CZ_P/2, Cm_P/2, Cn_P/2, Cl_P/2
  alpha/1 -> Alpha Lookup/1
  CY_P/1 -> Gain5/1
  CZ_P/1 -> Gain3/1
  Cl_P/1 -> Mux/4
  Cn_P/1 -> Mux/6
  Mux/1 -> coefficients/1
  Gain/1 -> Mux/2
  Cm_P/1 -> Gain2/1
  Gain1/1 -> Mux/1
  Gain2/1 -> Gain4/1
  Gain3/1 -> Mux/3
  Gain4/1 -> Mux/5
  Gain5/1 -> Gain/1

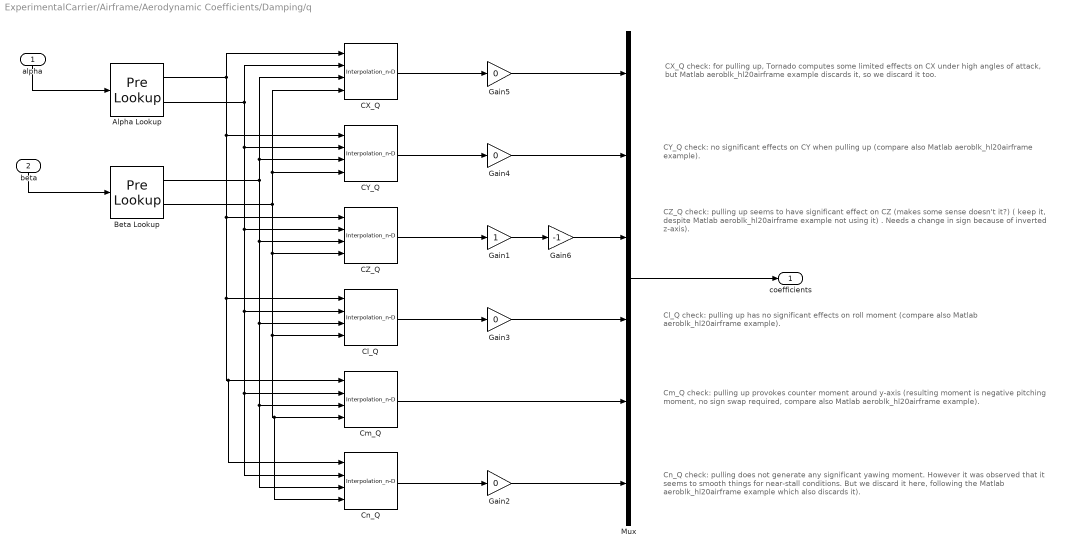
== system ExperimentalCarrier/Airframe/Aerodynamic Coefficients/Damping/q ==
  note: CX_Q check: for pulling up, Tornado computes some limited effects on CX under high angles of attack, but Matlab aeroblk_hl20airframe example discards it, so we discard it too.
  note: CZ_Q check: pulling up seems to have significant effect on CZ (makes some sense doesn't it?) ( keep it, despite Matlab aeroblk_hl20airframe example not using it) . Needs a change in sign because of inverted z-axis).
  note: Cl_Q check: pulling up has no significant effects on roll moment (compare also Matlab aeroblk_hl20airframe example).
  note: Cn_Q check: pulling does not generate any significant yawing moment. However it was observed that it seems to smooth things for near-stall conditions. But we discard it here, following the Matlab aeroblk_hl20airframe example which also discards it).
  note: Cm_Q check: pulling up provokes counter moment around y-axis (resulting moment is negative pitching moment, no sign swap required, compare also Matlab aeroblk_hl20airframe example).
  note: CY_Q check: no significant effects on CY when pulling up (compare also Matlab aeroblk_hl20airframe example).
  alpha : Inport
  beta : Inport  Port=2
  Alpha Lookup : PreLookup  BreakpointsData=alpha*180/pi  ExtrapMethod=Linear
  Beta Lookup : PreLookup  BreakpointsData=beta*180/pi  ExtrapMethod=Linear
  CX_Q : Interpolation_n-D  Table=CX_Q  InternalRulePriority=Speed
  CY_Q : Interpolation_n-D  Table=CY_Q  InternalRulePriority=Speed
  CZ_Q : Interpolation_n-D  Table=CZ_Q  InternalRulePriority=Speed
  Cl_Q : Interpolation_n-D  Table=Cl_Q  InternalRulePriority=Speed
  Cm_Q : Interpolation_n-D  Table=Cm_Q  InternalRulePriority=Speed
  Cn_Q : Interpolation_n-D  Table=Cn_Q  InternalRulePriority=Speed
  Gain1 : Gain
  Gain{2..5} (4 alike) : Gain  Gain=0
  Gain6 : Gain  Gain=-1
  Mux : Mux  Inputs=6
  coefficients : Outport
  wires:
  CZ_Q/1 -> Gain1/1
  Alpha Lookup/2 -> CY_Q/2, CZ_Q/2, Cn_Q/2, Cm_Q/2, Cl_Q/2, CX_Q/2
  CY_Q/1 -> Gain4/1
  Alpha Lookup/1 -> CY_Q/1, CZ_Q/1, Cl_Q/1, Cn_Q/1, Cm_Q/1, CX_Q/1
  Cm_Q/1 -> Mux/5
  beta/1 -> Beta Lookup/1
  Beta Lookup/1 -> Cn_Q/3, Cm_Q/3, Cl_Q/3, CZ_Q/3, CX_Q/3, CY_Q/3
  Beta Lookup/2 -> CY_Q/4, CX_Q/4, Cn_Q/4, Cm_Q/4, Cl_Q/4, CZ_Q/4
  Mux/1 -> coefficients/1
  alpha/1 -> Alpha Lookup/1
  CX_Q/1 -> Gain5/1
  Gain1/1 -> Gain6/1
  Cn_Q/1 -> Gain2/1
  Gain2/1 -> Mux/6
  Cl_Q/1 -> Gain3/1
  Gain3/1 -> Mux/4
  Gain4/1 -> Mux/2
  Gain5/1 -> Mux/1
  Gain6/1 -> Mux/3

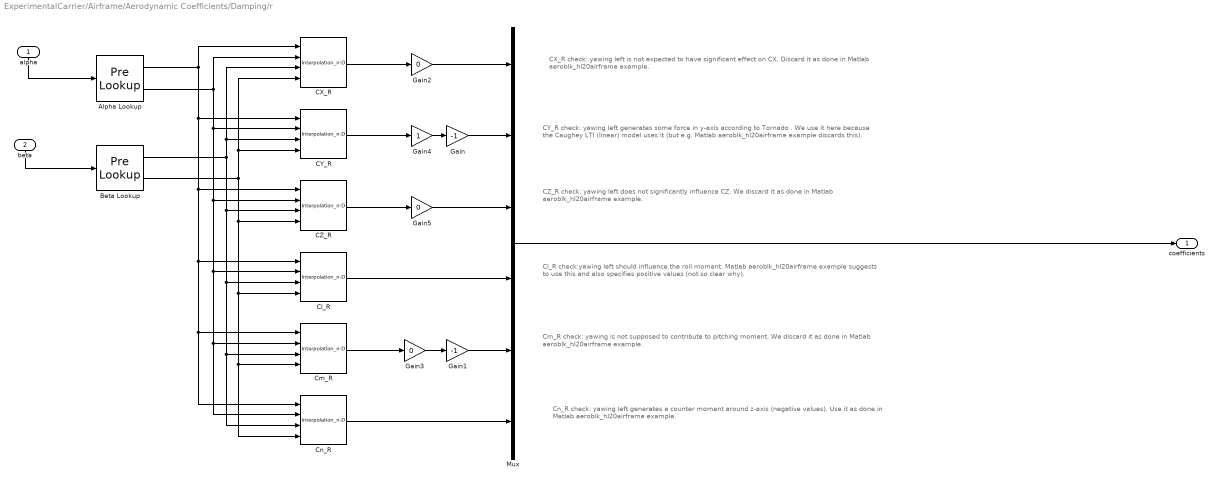
== system ExperimentalCarrier/Airframe/Aerodynamic Coefficients/Damping/r ==
  note: Cn_R check: yawing left generates a counter moment around z-axis (negative values). Use it as done in Matlab aeroblk_hl20airframe example.
  note: Cm_R check: yawing is not supposed to contribute to pitching moment. We discard it as done in Matlab aeroblk_hl20airframe example.
  note: Cl_R check:yawing left should influence the roll moment. Matlab aeroblk_hl20airframe example suggests to use this and also specifies positive values (not so clear why).
  note: CZ_R check: yawing left does not significantly influence CZ. We discard it as done in Matlab aeroblk_hl20airframe example.
  note: CY_R check: yawing left generates some force in y-axis according to Tornado . We use it here
      | because the Caughey LTI (linear) model uses it (but e.g. Matlab aeroblk_hl20airframe example discards this).
  note: CX_R check: yawing left is not expected to have significant effect on CX. Discard it as done in Matlab aeroblk_hl20airframe example.
  alpha : Inport
  beta : Inport  Port=2
  Alpha Lookup : PreLookup  BreakpointsData=alpha*180/pi  ExtrapMethod=Linear
  Beta Lookup : PreLookup  BreakpointsData=beta*180/pi  ExtrapMethod=Linear
  CX_R : Interpolation_n-D  Table=CX_R  InternalRulePriority=Speed
  CY_R : Interpolation_n-D  Table=CY_R  InternalRulePriority=Speed
  CZ_R : Interpolation_n-D  Table=CZ_R  InternalRulePriority=Speed
  Cl_R : Interpolation_n-D  Table=Cl_R  InternalRulePriority=Speed
  Cm_R : Interpolation_n-D  Table=Cm_R  InternalRulePriority=Speed
  Cn_R : Interpolation_n-D  Table=Cn_R  InternalRulePriority=Speed
  Gain : Gain  Gain=-1
  Gain1 : Gain  Gain=-1
  Gain2 : Gain  Gain=0
  Gain3 : Gain  Gain=0
  Gain4 : Gain
  Gain5 : Gain  Gain=0
  Mux : Mux  Inputs=6
  coefficients : Outport
  wires:
  CZ_R/1 -> Gain5/1
  Alpha Lookup/2 -> CY_R/2, CZ_R/2, Cm_R/2, Cn_R/2, Cl_R/2, CX_R/2
  CY_R/1 -> Gain4/1
  Alpha Lookup/1 -> CX_R/1, CY_R/1, CZ_R/1, Cn_R/1, Cm_R/1, Cl_R/1
  Cm_R/1 -> Gain3/1
  Cl_R/1 -> Mux/4
  beta/1 -> Beta Lookup/1
  Beta Lookup/1 -> Cn_R/3, Cm_R/3, Cl_R/3, CZ_R/3, CY_R/3, CX_R/3
  Beta Lookup/2 -> Cn_R/4, Cm_R/4, Cl_R/4, CZ_R/4, CY_R/4, CX_R/4
  Cn_R/1 -> Mux/6
  Mux/1 -> coefficients/1
  alpha/1 -> Alpha Lookup/1
  CX_R/1 -> Gain2/1
  Gain/1 -> Mux/2
  Gain1/1 -> Mux/5
  Gain2/1 -> Mux/1
  Gain3/1 -> Gain1/1
  Gain4/1 -> Gain/1
  Gain5/1 -> Mux/3
